simulink model "PID_Controller"  (R2020b)
settings: Solver=VariableStepAuto  StartTime=0.0  StopTime=10.0  RelTol=1e-3
settings Model: Creator=mluser  LastModifiedBy=mluser

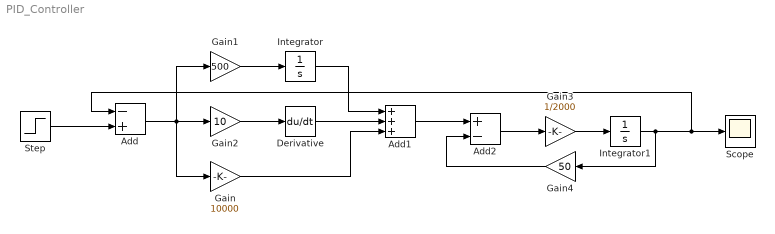
== system PID_Controller ==
  Add : Sum  Inputs=-+
  Add1 : Sum  Inputs=+++
  Add2 : Sum  Inputs=+-
  Derivative : Derivative  CoefficientInTFapproximation=1
  Gain : Gain  Gain=10000
  Gain1 : Gain  Gain=500
  Gain2 : Gain  Gain=10
  Gain3 : Gain  Gain=1/2000
  Gain4 : Gain  Gain=50
  Integrator : Integrator
  Integrator1 : Integrator
  Scope : Scope
  Step : Step  SampleTime=0
  wires:
  Add/1 -> Gain/1, Gain1/1, Gain2/1
  Step/1 -> Add/2
  Gain2/1 -> Derivative/1
  Gain1/1 -> Integrator/1
  Integrator/1 -> Add1/1
  Derivative/1 -> Add1/2
  Gain/1 -> Add1/3
  Add1/1 -> Add2/1
  Add2/1 -> Gain3/1
  Gain3/1 -> Integrator1/1
  Integrator1/1 -> Gain4/1, Add/1, Scope/1
  Gain4/1 -> Add2/2
